simulink model "ABS_virtual_no_fliter_40_88"  (R2023a)
settings: Solver=VariableStepAuto  StartTime=0.0  StopTime=inf  FixedStep=0.001  RelTol=1e-3  EnableMultiTasking=on
PreLoadFcn:
  | SoftABS_params
libraries: CarMaker4SL x28, simulink x19, dspsigops x5
(part 3 of 3)

== system ABS_virtual_no_fliter_40_88/CarMaker/IPG Vehicle/CarAndTrailer/Trailer/CreateBus Vhcl.Steering ==
  In1 : Inport
  Bus Creator3 : BusCreator  Inputs=4
  Demux : Demux
      settings: DisplayOption=none
  Out1 : Outport  VectorParamsAs1DForOutWhenUnconnected=off
  wires:
  Bus Creator3/1 -> Out1/1
  Demux/1 -> Bus Creator3/1  "Vhcl Steering Ang"
  Demux/3 -> Bus Creator3/3  "Vhcl Steering AngAcc"
  Demux/2 -> Bus Creator3/2  "Vhcl Steering AngVel"
  Demux/4 -> Bus Creator3/4  "Vhcl Steering Trq"
  In1/1 -> Demux/1

== system ABS_virtual_no_fliter_40_88/CarMaker/IPG Vehicle/CarAndTrailer/Trailer/CreateBus Vhcl.Wheel.FL ==
  In1 : Inport
  Bus Creator3 : BusCreator  Inputs=14
  Demux3 : Demux  Outputs=14
      settings: DisplayOption=none
  Out1 : Outport  VectorParamsAs1DForOutWhenUnconnected=off
  wires:
  Demux3/14 -> Bus Creator3/14  "Vhcl Wheel FL Trq_WhlBearing"
  Demux3/13 -> Bus Creator3/13  "Vhcl Wheel FL Trq_T2W"
  Demux3/12 -> Bus Creator3/12  "Vhcl Wheel FL SideSlip"
  Demux3/11 -> Bus Creator3/11  "Vhcl Wheel FL LongSlip"
  Demux3/10 -> Bus Creator3/10  "Vhcl Wheel FL vBelt"
  Demux3/9 -> Bus Creator3/9  "Vhcl Wheel FL Fz"
  Demux3/8 -> Bus Creator3/8  "Vhcl Wheel FL Fy"
  Demux3/7 -> Bus Creator3/7  "Vhcl Wheel FL Fx"
  Demux3/6 -> Bus Creator3/6  "Vhcl Wheel FL r_zxy z"
  Demux3/5 -> Bus Creator3/5  "Vhcl Wheel FL r_zxy y"
  Demux3/4 -> Bus Creator3/4  "Vhcl Wheel FL r_zxy x"
  Demux3/3 -> Bus Creator3/3  "Vhcl Wheel FL t z"
  Demux3/2 -> Bus Creator3/2  "Vhcl Wheel FL t y"
  In1/1 -> Demux3/1
  Bus Creator3/1 -> Out1/1
  Demux3/1 -> Bus Creator3/1  "Vhcl Wheel FL t x"

== system ABS_virtual_no_fliter_40_88/CarMaker/IPG Vehicle/CarAndTrailer/Trailer/CreateBus Vhcl.Wheel.FR ==
  In1 : Inport
  Bus Creator3 : BusCreator  Inputs=14
  Demux3 : Demux  Outputs=14
      settings: DisplayOption=none
  Out1 : Outport  VectorParamsAs1DForOutWhenUnconnected=off
  wires:
  Demux3/14 -> Bus Creator3/14  "Vhcl Wheel FR Trq_WhlBearing"
  Demux3/13 -> Bus Creator3/13  "Vhcl Wheel FR Trq_T2W"
  Demux3/12 -> Bus Creator3/12  "Vhcl Wheel FR SideSlip"
  Demux3/11 -> Bus Creator3/11  "Vhcl Wheel FR LongSlip"
  Demux3/10 -> Bus Creator3/10  "Vhcl Wheel FR vBelt"
  Demux3/9 -> Bus Creator3/9  "Vhcl Wheel FR Fz"
  Demux3/8 -> Bus Creator3/8  "Vhcl Wheel FR Fy"
  Demux3/7 -> Bus Creator3/7  "Vhcl Wheel FR Fx"
  Demux3/6 -> Bus Creator3/6  "Vhcl Wheel FR r_zxy z"
  Demux3/5 -> Bus Creator3/5  "Vhcl Wheel FR r_zxy y"
  Demux3/4 -> Bus Creator3/4  "Vhcl Wheel FR r_zxy x"
  Demux3/3 -> Bus Creator3/3  "Vhcl Wheel FR t z"
  Demux3/2 -> Bus Creator3/2  "Vhcl Wheel FR t y"
  In1/1 -> Demux3/1
  Bus Creator3/1 -> Out1/1
  Demux3/1 -> Bus Creator3/1  "Vhcl Wheel FR t x"

== system ABS_virtual_no_fliter_40_88/CarMaker/IPG Vehicle/CarAndTrailer/Trailer/CreateBus Vhcl.Wheel.RL ==
  In1 : Inport
  Bus Creator3 : BusCreator  Inputs=14
  Demux3 : Demux  Outputs=14
      settings: DisplayOption=none
  Out1 : Outport  VectorParamsAs1DForOutWhenUnconnected=off
  wires:
  Demux3/14 -> Bus Creator3/14  "Vhcl Wheel RL Trq_WhlBearing"
  Demux3/13 -> Bus Creator3/13  "Vhcl Wheel RL Trq_T2W"
  Demux3/12 -> Bus Creator3/12  "Vhcl Wheel RL SideSlip"
  Demux3/11 -> Bus Creator3/11  "Vhcl Wheel RL LongSlip"
  Demux3/10 -> Bus Creator3/10  "Vhcl Wheel RL vBelt"
  Demux3/9 -> Bus Creator3/9  "Vhcl Wheel RL Fz"
  Demux3/8 -> Bus Creator3/8  "Vhcl Wheel RL Fy"
  Demux3/7 -> Bus Creator3/7  "Vhcl Wheel RL Fx"
  Demux3/6 -> Bus Creator3/6  "Vhcl Wheel RL r_zxy z"
  Demux3/5 -> Bus Creator3/5  "Vhcl Wheel RL r_zxy y"
  Demux3/4 -> Bus Creator3/4  "Vhcl Wheel RL r_zxy x"
  Demux3/3 -> Bus Creator3/3  "Vhcl Wheel RL t z"
  Demux3/2 -> Bus Creator3/2  "Vhcl Wheel RL t y"
  In1/1 -> Demux3/1
  Bus Creator3/1 -> Out1/1
  Demux3/1 -> Bus Creator3/1  "Vhcl Wheel RL t x"

== system ABS_virtual_no_fliter_40_88/CarMaker/IPG Vehicle/CarAndTrailer/Trailer/CreateBus Vhcl.Wheel.RR ==
  In1 : Inport
  Bus Creator3 : BusCreator  Inputs=14
  Demux3 : Demux  Outputs=14
      settings: DisplayOption=none
  Out1 : Outport  VectorParamsAs1DForOutWhenUnconnected=off
  wires:
  Demux3/14 -> Bus Creator3/14  "Vhcl Wheel RR Trq_WhlBearing"
  Demux3/13 -> Bus Creator3/13  "Vhcl Wheel RR Trq_T2W"
  Demux3/12 -> Bus Creator3/12  "Vhcl Wheel RR SideSlip"
  Demux3/11 -> Bus Creator3/11  "Vhcl Wheel RR LongSlip"
  Demux3/10 -> Bus Creator3/10  "Vhcl Wheel RR vBelt"
  Demux3/9 -> Bus Creator3/9  "Vhcl Wheel RR Fz"
  Demux3/8 -> Bus Creator3/8  "Vhcl Wheel RR Fy"
  Demux3/7 -> Bus Creator3/7  "Vhcl Wheel RR Fx"
  Demux3/6 -> Bus Creator3/6  "Vhcl Wheel RR r_zxy z"
  Demux3/5 -> Bus Creator3/5  "Vhcl Wheel RR r_zxy y"
  Demux3/4 -> Bus Creator3/4  "Vhcl Wheel RR r_zxy x"
  Demux3/3 -> Bus Creator3/3  "Vhcl Wheel RR t z"
  Demux3/2 -> Bus Creator3/2  "Vhcl Wheel RR t y"
  In1/1 -> Demux3/1
  Bus Creator3/1 -> Out1/1
  Demux3/1 -> Bus Creator3/1  "Vhcl Wheel RR t x"

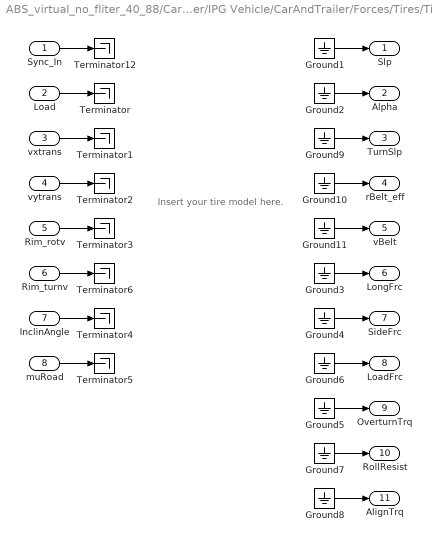
== system ABS_virtual_no_fliter_40_88/CarMaker/IPG Vehicle/CarAndTrailer/Forces/Tires/TireFL ==
  note: Insert your tire model here.
  Sync_In : Inport
  Load : Inport  Port=2
  vxtrans : Inport  Port=3
  vytrans : Inport  Port=4
  Rim_rotv : Inport  Port=5
  Rim_turnv : Inport  Port=6
  InclinAngle : Inport  Port=7
  muRoad : Inport  Port=8
  Ground{1..11} (11 alike) : Ground
  Terminator{,1..6,12} (8 alike) : Terminator
  Slp : Outport  VectorParamsAs1DForOutWhenUnconnected=off
  Alpha : Outport  Port=2  VectorParamsAs1DForOutWhenUnconnected=off
  TurnSlp : Outport  Port=3  VectorParamsAs1DForOutWhenUnconnected=off
  rBelt_eff : Outport  Port=4  VectorParamsAs1DForOutWhenUnconnected=off
  vBelt : Outport  Port=5  VectorParamsAs1DForOutWhenUnconnected=off
  LongFrc : Outport  Port=6  VectorParamsAs1DForOutWhenUnconnected=off
  SideFrc : Outport  Port=7  VectorParamsAs1DForOutWhenUnconnected=off
  LoadFrc : Outport  Port=8  VectorParamsAs1DForOutWhenUnconnected=off
  OverturnTrq : Outport  Port=9  VectorParamsAs1DForOutWhenUnconnected=off
  RollResist : Outport  Port=10  VectorParamsAs1DForOutWhenUnconnected=off
  AlignTrq : Outport  Port=11  VectorParamsAs1DForOutWhenUnconnected=off
  wires:
  Ground11/1 -> vBelt/1
  Ground10/1 -> rBelt_eff/1
  Ground9/1 -> TurnSlp/1
  Rim_turnv/1 -> Terminator6/1
  Sync_In/1 -> Terminator12/1
  Ground2/1 -> Alpha/1
  Ground3/1 -> LongFrc/1
  Ground4/1 -> SideFrc/1
  Ground5/1 -> OverturnTrq/1
  vxtrans/1 -> Terminator1/1
  vytrans/1 -> Terminator2/1
  Rim_rotv/1 -> Terminator3/1
  InclinAngle/1 -> Terminator4/1
  muRoad/1 -> Terminator5/1
  Load/1 -> Terminator/1
  Ground1/1 -> Slp/1
  Ground6/1 -> LoadFrc/1
  Ground7/1 -> RollResist/1
  Ground8/1 -> AlignTrq/1

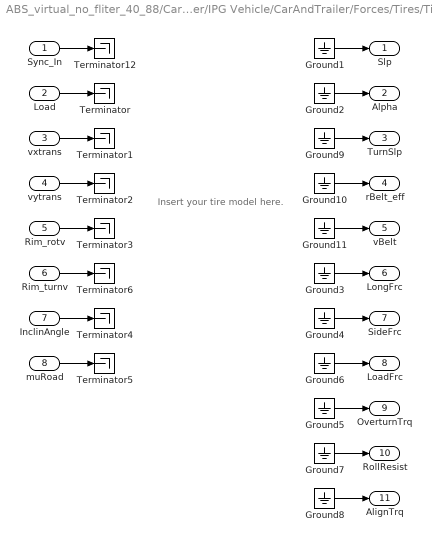
== system ABS_virtual_no_fliter_40_88/CarMaker/IPG Vehicle/CarAndTrailer/Forces/Tires/TireFR ==
  note: Insert your tire model here.
  Sync_In : Inport
  Load : Inport  Port=2
  vxtrans : Inport  Port=3
  vytrans : Inport  Port=4
  Rim_rotv : Inport  Port=5
  Rim_turnv : Inport  Port=6
  InclinAngle : Inport  Port=7
  muRoad : Inport  Port=8
  Ground{1..11} (11 alike) : Ground
  Terminator{,1..6,12} (8 alike) : Terminator
  Slp : Outport  VectorParamsAs1DForOutWhenUnconnected=off
  Alpha : Outport  Port=2  VectorParamsAs1DForOutWhenUnconnected=off
  TurnSlp : Outport  Port=3  VectorParamsAs1DForOutWhenUnconnected=off
  rBelt_eff : Outport  Port=4  VectorParamsAs1DForOutWhenUnconnected=off
  vBelt : Outport  Port=5  VectorParamsAs1DForOutWhenUnconnected=off
  LongFrc : Outport  Port=6  VectorParamsAs1DForOutWhenUnconnected=off
  SideFrc : Outport  Port=7  VectorParamsAs1DForOutWhenUnconnected=off
  LoadFrc : Outport  Port=8  VectorParamsAs1DForOutWhenUnconnected=off
  OverturnTrq : Outport  Port=9  VectorParamsAs1DForOutWhenUnconnected=off
  RollResist : Outport  Port=10  VectorParamsAs1DForOutWhenUnconnected=off
  AlignTrq : Outport  Port=11  VectorParamsAs1DForOutWhenUnconnected=off
  wires:
  Ground11/1 -> vBelt/1
  Ground10/1 -> rBelt_eff/1
  Ground9/1 -> TurnSlp/1
  Rim_turnv/1 -> Terminator6/1
  Sync_In/1 -> Terminator12/1
  Ground2/1 -> Alpha/1
  Ground3/1 -> LongFrc/1
  Ground4/1 -> SideFrc/1
  Ground5/1 -> OverturnTrq/1
  vxtrans/1 -> Terminator1/1
  vytrans/1 -> Terminator2/1
  Rim_rotv/1 -> Terminator3/1
  InclinAngle/1 -> Terminator4/1
  muRoad/1 -> Terminator5/1
  Load/1 -> Terminator/1
  Ground1/1 -> Slp/1
  Ground6/1 -> LoadFrc/1
  Ground7/1 -> RollResist/1
  Ground8/1 -> AlignTrq/1

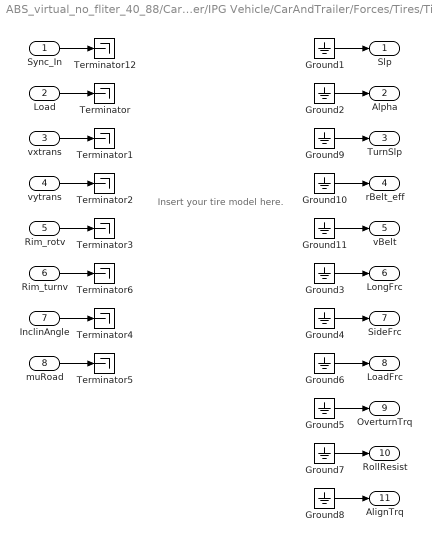
== system ABS_virtual_no_fliter_40_88/CarMaker/IPG Vehicle/CarAndTrailer/Forces/Tires/TireRL ==
  note: Insert your tire model here.
  Sync_In : Inport
  Load : Inport  Port=2
  vxtrans : Inport  Port=3
  vytrans : Inport  Port=4
  Rim_rotv : Inport  Port=5
  Rim_turnv : Inport  Port=6
  InclinAngle : Inport  Port=7
  muRoad : Inport  Port=8
  Ground{1..11} (11 alike) : Ground
  Terminator{,1..6,12} (8 alike) : Terminator
  Slp : Outport  VectorParamsAs1DForOutWhenUnconnected=off
  Alpha : Outport  Port=2  VectorParamsAs1DForOutWhenUnconnected=off
  TurnSlp : Outport  Port=3  VectorParamsAs1DForOutWhenUnconnected=off
  rBelt_eff : Outport  Port=4  VectorParamsAs1DForOutWhenUnconnected=off
  vBelt : Outport  Port=5  VectorParamsAs1DForOutWhenUnconnected=off
  LongFrc : Outport  Port=6  VectorParamsAs1DForOutWhenUnconnected=off
  SideFrc : Outport  Port=7  VectorParamsAs1DForOutWhenUnconnected=off
  LoadFrc : Outport  Port=8  VectorParamsAs1DForOutWhenUnconnected=off
  OverturnTrq : Outport  Port=9  VectorParamsAs1DForOutWhenUnconnected=off
  RollResist : Outport  Port=10  VectorParamsAs1DForOutWhenUnconnected=off
  AlignTrq : Outport  Port=11  VectorParamsAs1DForOutWhenUnconnected=off
  wires:
  Ground11/1 -> vBelt/1
  Ground10/1 -> rBelt_eff/1
  Ground9/1 -> TurnSlp/1
  Rim_turnv/1 -> Terminator6/1
  Sync_In/1 -> Terminator12/1
  Ground2/1 -> Alpha/1
  Ground3/1 -> LongFrc/1
  Ground4/1 -> SideFrc/1
  Ground5/1 -> OverturnTrq/1
  vxtrans/1 -> Terminator1/1
  vytrans/1 -> Terminator2/1
  Rim_rotv/1 -> Terminator3/1
  InclinAngle/1 -> Terminator4/1
  muRoad/1 -> Terminator5/1
  Load/1 -> Terminator/1
  Ground1/1 -> Slp/1
  Ground6/1 -> LoadFrc/1
  Ground7/1 -> RollResist/1
  Ground8/1 -> AlignTrq/1

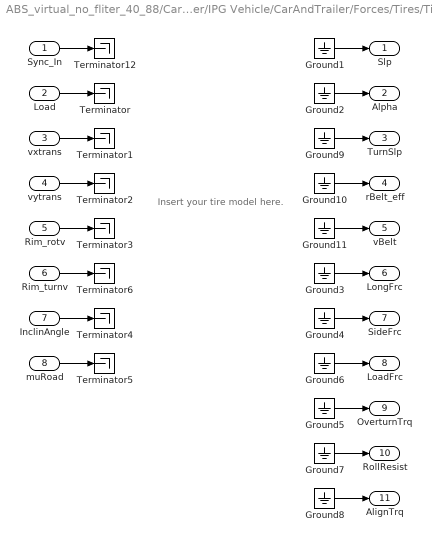
== system ABS_virtual_no_fliter_40_88/CarMaker/IPG Vehicle/CarAndTrailer/Forces/Tires/TireRR ==
  note: Insert your tire model here.
  Sync_In : Inport
  Load : Inport  Port=2
  vxtrans : Inport  Port=3
  vytrans : Inport  Port=4
  Rim_rotv : Inport  Port=5
  Rim_turnv : Inport  Port=6
  InclinAngle : Inport  Port=7
  muRoad : Inport  Port=8
  Ground{1..11} (11 alike) : Ground
  Terminator{,1..6,12} (8 alike) : Terminator
  Slp : Outport  VectorParamsAs1DForOutWhenUnconnected=off
  Alpha : Outport  Port=2  VectorParamsAs1DForOutWhenUnconnected=off
  TurnSlp : Outport  Port=3  VectorParamsAs1DForOutWhenUnconnected=off
  rBelt_eff : Outport  Port=4  VectorParamsAs1DForOutWhenUnconnected=off
  vBelt : Outport  Port=5  VectorParamsAs1DForOutWhenUnconnected=off
  LongFrc : Outport  Port=6  VectorParamsAs1DForOutWhenUnconnected=off
  SideFrc : Outport  Port=7  VectorParamsAs1DForOutWhenUnconnected=off
  LoadFrc : Outport  Port=8  VectorParamsAs1DForOutWhenUnconnected=off
  OverturnTrq : Outport  Port=9  VectorParamsAs1DForOutWhenUnconnected=off
  RollResist : Outport  Port=10  VectorParamsAs1DForOutWhenUnconnected=off
  AlignTrq : Outport  Port=11  VectorParamsAs1DForOutWhenUnconnected=off
  wires:
  Ground11/1 -> vBelt/1
  Ground10/1 -> rBelt_eff/1
  Ground9/1 -> TurnSlp/1
  Rim_turnv/1 -> Terminator6/1
  Sync_In/1 -> Terminator12/1
  Ground2/1 -> Alpha/1
  Ground3/1 -> LongFrc/1
  Ground4/1 -> SideFrc/1
  Ground5/1 -> OverturnTrq/1
  vxtrans/1 -> Terminator1/1
  vytrans/1 -> Terminator2/1
  Rim_rotv/1 -> Terminator3/1
  InclinAngle/1 -> Terminator4/1
  muRoad/1 -> Terminator5/1
  Load/1 -> Terminator/1
  Ground1/1 -> Slp/1
  Ground6/1 -> LoadFrc/1
  Ground7/1 -> RollResist/1
  Ground8/1 -> AlignTrq/1

== stateflow chart ABS_virtual_no_fliter_40_88/CarMaker/IPG Vehicle/Brake/SoftABS/ABS_RL/Chart_RL ==
  state ready
  state ABS_off
    entry, during:
    phase=0;
    pressure_state=4;
  state ABS_end
    entry:
    phase=0;
    pressure_state=4;
  state phase1
    entry, during:
    phase=1;
    pressure_state=4;
  state phase2
    entry, during:
    phase=2;
    pressure_state=1;
  state phase3
    entry, during:
    phase=3;
    pressure_state=3;
  state phase4
    entry, during:
    phase=4;
    pressure_state=1;
  state phase5
    entry, during:
    phase=5;
    pressure_state=2;
  state phase6
    entry, during:
    phase=6;
    pressure_state=1;
  state phase7
    entry, during:
    phase=7;
    pressure_state=2;
  (default) -> ready
  ready -> ABS_off : [b_trq_in>=(b_trq_min+1)]
  ABS_end -> (junction 873) : [(slip>0.07)]
  ABS_off -> (junction 868) [order 2] : [slip>slip_switch]
  (junction 873) -> (junction 863)
  (junction 868) -> (junction 869)
  ABS_off -> phase1 [order 1] : [(whl_a<0)&&(b_trq_in>=b_trq_min)&&(slip>=slip_switch)]
  (junction 883) -> ABS_end
  phase1 -> phase2 : [(whl_a<whl_a_min)]
  phase2 -> phase3 : [v_whl<v_whl_switch]
  (junction 869) -> phase3
  (junction 878) -> (junction 869)
  phase3 -> (junction 883) [order 2] : [(slip<0.001)&&(deceleration_rate<0.5)&&(v_car<=1.5)&&(whl_a>whl_a_min)]
  (junction 905) -> (junction 883)
  (junction 863) -> phase3
  (junction 906) -> phase3
  (junction 858) -> (junction 906) [order 2]
  phase3 -> phase4 [order 1] : [whl_a>(whl_a_min)]
  (junction 858) -> (junction 905) [order 1] : [(v_car<=5)]
  (junction 888) -> (junction 858)
  (junction 865) -> (junction 905)
  phase4 -> (junction 888) [order 2] : [(whl_a<whl_a_min)&&(slip>slip_switch)]
  phase4 -> (junction 865) [commented out] : [(slip<0.001)&&(deceleration_rate<5)]
  (junction 887) -> (junction 865)
  phase4 -> phase5 [order 1] : [whl_a>10*(whl_a_max)]
  phase5 -> (junction 887) [commented out] : [(slip<0.001)&&(deceleration_rate<5)]
  (junction 894) -> (junction 887)
  phase5 -> phase6 : [whl_a<10*(whl_a_max)]
  phase6 -> (junction 894) [commented out] : [(slip<0.001)&&(deceleration_rate<5)]
  (junction 882) -> (junction 894)
  phase6 -> phase7 : [whl_a<whl_a_max]
  phase7 -> (junction 878) [order 1] : [(whl_a<whl_a_min)&&(v_whl<v_whl_switch)&&(slip>slip_switch)]
  phase7 -> (junction 882) [order 2] : [(slip<0.001)&&(deceleration_rate<0.5)&&(v_car<=1.5)&&(whl_a>whl_a_min)]
  data: b_trq_in input; slip input; b_trq_min input; pressure_state output; phase output; slip_switch input; v_whl input; v_whl_switch input; whl_a input; whl_a_max input; whl_a_min input; deceleration_rate input; v_car input

== stateflow chart ABS_virtual_no_fliter_40_88/CarMaker/IPG Vehicle/Brake/SoftABS/ABS_FL/Chart_FL ==
  state ready
  state ABS_off
    entry, during:
    phase=0;
    pressure_state=4;
  state ABS_end
    entry:
    phase=0;
    pressure_state=4;
  state phase1
    entry, during:
    phase=1;
    pressure_state=4;
  state phase2
    entry, during:
    phase=2;
    pressure_state=1;
  state phase3
    entry, during:
    phase=3;
    pressure_state=3;
  state phase4
    entry, during:
    phase=4;
    pressure_state=1;
  state phase5
    entry, during:
    phase=5;
    pressure_state=2;
  state phase6
    entry, during:
    phase=6;
    pressure_state=1;
  state phase7
    entry, during:
    phase=7;
    pressure_state=2;
  (default) -> ready
  ready -> ABS_off : [b_trq_in>=(b_trq_min+1)]
  ABS_end -> (junction 786) : [(slip>0.07)]
  ABS_off -> (junction 781) [order 2] : [slip>slip_switch]
  (junction 786) -> (junction 776)
  (junction 781) -> (junction 782)
  ABS_off -> phase1 [order 1] : [(whl_a<0)&&(b_trq_in>=b_trq_min)&&(slip>=slip_switch)]
  (junction 796) -> ABS_end
  phase1 -> phase2 : [(whl_a<whl_a_min)]
  phase2 -> phase3 : [v_whl<v_whl_switch]
  (junction 782) -> phase3
  (junction 791) -> (junction 782)
  phase3 -> (junction 796) [order 2] : [(slip<0.001)&&(deceleration_rate<0.5)&&(v_car<=1.5)&&(whl_a>whl_a_min)]
  (junction 818) -> (junction 796)
  (junction 776) -> phase3
  (junction 819) -> phase3
  (junction 771) -> (junction 819) [order 2]
  phase3 -> phase4 [order 1] : [whl_a>(whl_a_min)]
  (junction 771) -> (junction 818) [order 1] : [(v_car<=5)]
  (junction 801) -> (junction 771)
  (junction 778) -> (junction 818)
  phase4 -> (junction 801) [order 2] : [(whl_a<whl_a_min)&&(slip>slip_switch)]
  phase4 -> (junction 778) [commented out] : [(slip<0.001)&&(deceleration_rate<5)]
  (junction 800) -> (junction 778)
  phase4 -> phase5 [order 1] : [whl_a>10*(whl_a_max)]
  phase5 -> (junction 800) [commented out] : [(slip<0.001)&&(deceleration_rate<5)]
  (junction 807) -> (junction 800)
  phase5 -> phase6 : [whl_a<10*(whl_a_max)]
  phase6 -> (junction 807) [commented out] : [(slip<0.001)&&(deceleration_rate<5)]
  (junction 795) -> (junction 807)
  phase6 -> phase7 : [whl_a<whl_a_max]
  phase7 -> (junction 791) [order 1] : [(whl_a<whl_a_min)&&(v_whl<v_whl_switch)&&(slip>slip_switch)]
  phase7 -> (junction 795) [order 2] : [(slip<0.001)&&(deceleration_rate<0.5)&&(v_car<=1.5)&&(whl_a>whl_a_min)]
  data: b_trq_in input; slip input; b_trq_min input; pressure_state output; phase output; slip_switch input; v_whl input; v_whl_switch input; whl_a input; whl_a_max input; whl_a_min input; deceleration_rate input; v_car input

== stateflow chart ABS_virtual_no_fliter_40_88/CarMaker/IPG Vehicle/Brake/SoftABS/ABS_RR/Chart_RR ==
  state ready
  state ABS_off
    entry, during:
    phase=0;
    pressure_state=4;
  state ABS_end
    entry:
    phase=0;
    pressure_state=4;
  state phase1
    entry, during:
    phase=1;
    pressure_state=4;
  state phase2
    entry, during:
    phase=2;
    pressure_state=1;
  state phase3
    entry, during:
    phase=3;
    pressure_state=3;
  state phase4
    entry, during:
    phase=4;
    pressure_state=1;
  state phase5
    entry, during:
    phase=5;
    pressure_state=2;
  state phase6
    entry, during:
    phase=6;
    pressure_state=1;
  state phase7
    entry, during:
    phase=7;
    pressure_state=2;
  (default) -> ready
  ready -> ABS_off : [b_trq_in>=(b_trq_min+1)]
  ABS_end -> (junction 819) : [(slip>0.07)]
  ABS_off -> (junction 826) [order 2] : [slip>slip_switch]
  (junction 819) -> (junction 823)
  (junction 826) -> (junction 805)
  ABS_off -> phase1 [order 1] : [(whl_a<0)&&(b_trq_in>=b_trq_min)&&(slip>=slip_switch)]
  (junction 828) -> ABS_end
  phase1 -> phase2 : [(whl_a<whl_a_min)]
  phase2 -> phase3 : [v_whl<v_whl_switch]
  (junction 805) -> phase3
  (junction 795) -> (junction 805)
  phase3 -> (junction 828) [order 2] : [(slip<0.001)&&(deceleration_rate<0.5)&&(v_car<=1.5)&&(whl_a>whl_a_min)]
  (junction 840) -> (junction 828)
  (junction 823) -> phase3
  (junction 851) -> phase3
  (junction 842) -> (junction 851) [order 2]
  phase3 -> phase4 [order 1] : [whl_a>(whl_a_min)]
  (junction 842) -> (junction 840) [order 1] : [(v_car<=5)]
  (junction 830) -> (junction 842)
  (junction 807) -> (junction 840)
  phase4 -> (junction 830) [order 2] : [(whl_a<whl_a_min)&&(slip>slip_switch)]
  phase4 -> (junction 807) [commented out] : [(slip<0.001)&&(deceleration_rate<5)]
  (junction 825) -> (junction 807)
  phase4 -> phase5 [order 1] : [whl_a>10*(whl_a_max)]
  phase5 -> (junction 825) [commented out] : [(slip<0.001)&&(deceleration_rate<5)]
  (junction 800) -> (junction 825)
  phase5 -> phase6 : [whl_a<10*(whl_a_max)]
  phase6 -> (junction 800) [commented out] : [(slip<0.001)&&(deceleration_rate<5)]
  (junction 808) -> (junction 800)
  phase6 -> phase7 : [whl_a<whl_a_max]
  phase7 -> (junction 795) [order 1] : [(whl_a<whl_a_min)&&(v_whl<v_whl_switch)&&(slip>slip_switch)]
  phase7 -> (junction 808) [order 2] : [(slip<0.001)&&(deceleration_rate<0.5)&&(v_car<=1.5)&&(whl_a>whl_a_min)]
  data: b_trq_in input; slip input; b_trq_min input; pressure_state output; phase output; slip_switch input; v_whl input; v_whl_switch input; whl_a input; whl_a_max input; whl_a_min input; deceleration_rate input; v_car input

== stateflow chart ABS_virtual_no_fliter_40_88/CarMaker/IPG Vehicle/Brake/SoftABS/ABS_FR/Chart_FR ==
  state ready
  state ABS_off
    entry, during:
    phase=0;
    pressure_state=4;
  state ABS_end
    entry:
    phase=0;
    pressure_state=4;
  state phase1
    entry, during:
    phase=1;
    pressure_state=4;
  state phase2
    entry, during:
    phase=2;
    pressure_state=1;
  state phase3
    entry, during:
    phase=3;
    pressure_state=3;
  state phase4
    entry, during:
    phase=4;
    pressure_state=1;
  state phase5
    entry, during:
    phase=5;
    pressure_state=2;
  state phase6
    entry, during:
    phase=6;
    pressure_state=1;
  state phase7
    entry, during:
    phase=7;
    pressure_state=2;
  (default) -> ready
  ready -> ABS_off : [b_trq_in>=(b_trq_min+1)]
  ABS_end -> (junction 873) : [(slip>0.07)]
  ABS_off -> (junction 868) [order 2] : [slip>slip_switch]
  (junction 873) -> (junction 863)
  (junction 868) -> (junction 869)
  ABS_off -> phase1 [order 1] : [(whl_a<0)&&(b_trq_in>=b_trq_min)&&(slip>=slip_switch)]
  (junction 883) -> ABS_end
  phase1 -> phase2 : [(whl_a<whl_a_min)]
  phase2 -> phase3 : [v_whl<v_whl_switch]
  (junction 869) -> phase3
  (junction 878) -> (junction 869)
  phase3 -> (junction 883) [order 2] : [(slip<0.001)&&(deceleration_rate<0.5)&&(v_car<=1.5)&&(whl_a>whl_a_min)]
  (junction 905) -> (junction 883)
  (junction 863) -> phase3
  (junction 906) -> phase3
  (junction 858) -> (junction 906) [order 2]
  phase3 -> phase4 [order 1] : [whl_a>(whl_a_min)]
  (junction 858) -> (junction 905) [order 1] : [(v_car<=5)]
  (junction 888) -> (junction 858)
  (junction 865) -> (junction 905)
  phase4 -> (junction 888) [order 2] : [(whl_a<whl_a_min)&&(slip>slip_switch)]
  phase4 -> (junction 865) [commented out] : [(slip<0.001)&&(deceleration_rate<5)]
  (junction 887) -> (junction 865)
  phase4 -> phase5 [order 1] : [whl_a>10*(whl_a_max)]
  phase5 -> (junction 887) [commented out] : [(slip<0.001)&&(deceleration_rate<5)]
  (junction 894) -> (junction 887)
  phase5 -> phase6 : [whl_a<10*(whl_a_max)]
  phase6 -> (junction 894) [commented out] : [(slip<0.001)&&(deceleration_rate<5)]
  (junction 882) -> (junction 894)
  phase6 -> phase7 : [whl_a<whl_a_max]
  phase7 -> (junction 878) [order 1] : [(whl_a<whl_a_min)&&(v_whl<v_whl_switch)&&(slip>slip_switch)]
  phase7 -> (junction 882) [order 2] : [(slip<0.001)&&(deceleration_rate<0.5)&&(v_car<=1.5)&&(whl_a>whl_a_min)]
  data: b_trq_in input; slip input; b_trq_min input; pressure_state output; phase output; slip_switch input; v_whl input; v_whl_switch input; whl_a input; whl_a_max input; whl_a_min input; deceleration_rate input; v_car input
